simulink model "ES106A_StHlthSigStc"  (R2013b)
settings: Solver=FixedStepDiscrete  SolverMode=SingleTasking  StartTime=0.0  StopTime=1  FixedStep=0.002  RelTol=1e-3
undefined symbols (not defined in the file): APPL10_CNT_U08, BITSPERBYTE_CNT_U08, ENOTOK_CNT_U08, EOK_CNT_U08, LOWRMASKVAL_CNT_U32, NROFCRCAREA_CNT_U08, NVMAVRGPOSN_CNT_U08, NvmGetErrSts1, NVMMAXPOSN_CNT_U08, NVMMINPOSN_CNT_U08, NVMSAMPLECNTRPOSN_CNT_U08, RAMMAXPOSN_CNT_U08, RAMMINPOSN_CNT_U08, RAMRAWPOSN_CNT_U08, SIGCNT_ULS_U08, SigStcPrmInst, STHLTHMAXVAL_CNT_U08, STHLTHOSAPPL_CNT_U16, StHlthTaskRef1, WORDSIZE_CNT_U08
libraries: simulink x43, NxtrNvM x4, NxtrMax x4, NxtrMin x4, FloatToFixd x3, NxtrLim x2
(part 2 of 5)

== system ES106A_StHlthSigStc/StHlthSigStc/StHlthSigStcInit1/Check Applicability ==
  CalCRC8 : Inport
  Action Port : ActionPort  ActionType=then
  "Applicablity Check " : If  IfExpression=u1 == 1
  Constant : Constant  RequirementInfo={'linktype_rmi_doors' '0001022b (/ESG Group/FDD Module Requirements/EA4 Specific/ES106A_StHlthSigStc )' '#ES106A_48' 'true' 'REQ:ES106A_48' '' } %GIDa_4df2eb89_9649_4240_9516_a969529fb5fc  Value=0  OutDataTypeStr=uint8
      settings: AttributesFormatString=%<OutDataTypeStr>
  Data Store Read : DataStoreRead  DataStoreName=SigStcHistDataAry
  Do Nothing : Subsystem  TreatAsAtomicUnit=on
  Relational Operator : RelationalOperator  RequirementInfo={'linktype_rmi_doors' '0001022b (/ESG Group/FDD Module Requirements/EA4 Specific/ES106A_StHlthSigStc )' '#ES106A_50' 'true' 'REQ:ES106A_50' '' } %GIDa_be62b0a0_e56f_4259_a403_214fd52265b6  Operator=~=  OutDataTypeStr=boolean
  Selector : Selector  IndexMode=Zero-based  InputPortWidth=225  IndexOptions=Starting index (port)  Indices=[1 3]  OutputSizes=1
  Set Nvm Invalid : Subsystem  RequirementInfo={'linktype_rmi_doors' '0001022b (/ESG Group/FDD Module Requirements/EA4 Specific/ES106A_StHlthSigStc )' '#ES106A_44' 'true' 'REQ:ES106A_44' '' ; 'linktype_rmi_doors' '0001022b (/ESG Group/FDD Module Requirements/EA4 Specific/ES106A_StHlthSigStc )' '#ES106A_50' 'true' 'REQ:ES106A_50' '' } %GIDa_d83f31c6_88cf_451f_bc3f_a437a61baf7f  TreatAsAtomicUnit=on
  Subsystem5 : Subsystem  Description=|  mask(Copyright Information){none=on}
      | Copyright info block.                                               
      |                                                                     
      | Place copyright information at the top of every subsystem in design.
      mask prompts: none "No parameters"
      mask help: Place copyright information at the top of every subsystem in design.
      mask Display:
      | NxtrConf = 'Nexteer Confidential';
      | 
      | sys = bdroot; %handle for the current model ("system")
      | first = get_param(sys,'Created');
      | first = first(end-3:end);  %year is last four digits
      | 
      | last = get_param(sys,'LastModifiedDate');
      | if isempty(last)
      |     last = datestr(now,'yyyy');
      | else
      |     last = last(end-3:end);
      | end
      | 
      | if strcmp(first,last)
      |     fprintf('%s -- Copyright %s Nexteer',NxtrConf,first)
      | else
      |     fprintf('%s -- %s%s- %s Nexteer',NxtrConf,char(169),first,last)
      | end
  wires:
  CalCRC8/1 -> Relational Operator/2
  Relational Operator/1 -> "Applicablity Check "/1
  "Applicablity Check "/1 -> Set Nvm Invalid/Action
  "Applicablity Check "/2 -> Do Nothing/Action
  Data Store Read/1 -> Selector/1
  Constant/1 -> Selector/2
  Selector/1 -> Relational Operator/1

== system ES106A_StHlthSigStc/StHlthSigStc/StHlthSigStcInit1/CopyRight2 ==

== system ES106A_StHlthSigStc/StHlthSigStc/StHlthSigStcInit1/Crc_CalculateCRC8 ==
  note: This is the block representing the client call
  Crc_DataPtr : Inport
  Crc_Length : Inport  Port=2
  Crc_StartValue8 : Inport  Port=3
  Crc_IsFirstCall : Inport  Port=4
  Copyright1 : Subsystem  Description=|  mask(Copyright Information){none=on}
      | Copyright info block.                                               
      |                                                                     
      | Place copyright information at the top of every subsystem in design.
      mask prompts: none "No parameters"
      mask help: Place copyright information at the top of every subsystem in design.
      mask Display:
      | NxtrConf = 'Nexteer Confidential';
      | 
      | sys = bdroot; %handle for the current model ("system")
      | first = get_param(sys,'Created');
      | if(isempty(first))
      |     first = datestr(now,'yyyy');
      | else
      |     first = first(end-3:end);  %year is last four digits
      | end
      | 
      | last = get_param(sys,'LastModifiedDate');
      | if isempty(last)
      |     last = datestr(now,'yyyy');
      | else
      |     last = last(end-3:end);
      | end
      | 
      | if strcmp(first,last)
      |     fprintf('%s\nCopyright  %s Nexteer',NxtrConf,first);
      | else
      |     fprintf('%s\n%s%s-%s Nexteer',NxtrConf,char(169),first,last);
      | end
  FirstCall = False1 : Constant  Value=0  OutDataTypeStr=uint8
      settings: AttributesFormatString=%<OutDataTypeStr>
  FirstCall = False2 : Constant  Value=0  OutDataTypeStr=uint8
      settings: AttributesFormatString=%<OutDataTypeStr>
  Selector : Selector  IndexMode=Zero-based  InputPortWidth=32  IndexOptions=Starting index (port)  Indices=[1 3]  OutputSizes=1
  Terminator{1..4} (4 alike) : Terminator
  CalCRC8 : Outport
  wires:
  Crc_Length/1 -> Terminator1/1
  Crc_StartValue8/1 -> Terminator2/1
  Crc_IsFirstCall/1 -> Terminator3/1
  FirstCall = False1/1 -> CalCRC8/1
  Crc_DataPtr/1 -> Selector/1
  Selector/1 -> Terminator4/1
  FirstCall = False2/1 -> Selector/2

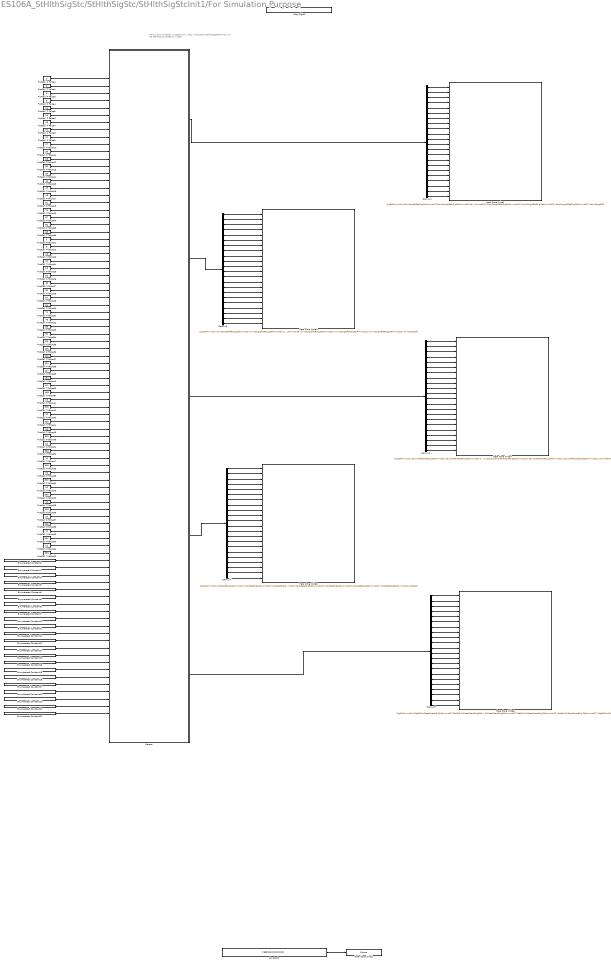
== system ES106A_StHlthSigStc/StHlthSigStc/StHlthSigStcInit1/For Simulation Purpose ==
  note: This is for Simulation purpose only.
      | Array of stucture 'StHlthSigStcPrmInst' will be defined as constant in code
  Constant9 : Constant  Description=[DUMMYAPPLCRC_CNT_U32 DUMMYCALL1CRC_CNT_U32 DUMMYCAL2CRC_CNT_U32 0 0 0 0 0]  Value=[100 10 0 0 0 0 0 0]  OutDataTypeStr=uint32
      settings: AttributesFormatString=%<Description>
  CopyRight2 : Subsystem  Description=|  mask(Copyright Information){none=on}
      | Copyright info block.                                               
      |                                                                     
      | Place copyright information at the top of every subsystem in design.
      mask prompts: none "No parameters"
      mask help: Place copyright information at the top of every subsystem in design.
      mask Display:
      | NxtrConf = 'Nexteer Confidential';
      | 
      | sys = bdroot; %handle for the current model ("system")
      | first = get_param(sys,'Created');
      | first = first(end-3:end);  %year is last four digits
      | 
      | last = get_param(sys,'LastModifiedDate');
      | if isempty(last)
      |     last = datestr(now,'yyyy');
      | else
      |     last = last(end-3:end);
      | end
      | 
      | if strcmp(first,last)
      |     fprintf('%s -- Copyright %s Nexteer',NxtrConf,first)
      | else
      |     fprintf('%s -- %s%s- %s Nexteer',NxtrConf,char(169),first,last)
      | end
  Data Store Write1 : DataStoreWrite  DataStoreName=CrcInst
  Data Store Write2 : DataStoreWrite  DataStoreName=SigStcPrmInst  DataStoreElements=SigStcPrmInst(1).RamStorgOffs#SigStcPrmInst(2).RamStorgOffs#SigStcPrmInst(3).RamStorgOffs#SigStcPrmInst(4).RamStorgOffs#SigStcPrmInst(5).RamStorgOffs#SigStcPrmInst(6).RamStorgOffs#SigStcPrmInst(7).RamStorgOffs#SigStcPrmInst(8).RamStorgOffs#SigStcPrmInst(9).RamStorgOffs#SigStcPrmInst(10).RamStorgOffs#SigStcPrmInst(11).RamStorgOffs#SigStcPrmInst(12).RamStorgOffs#SigStcPrmInst(13).RamStorgOffs#SigStcPrmInst(14).RamStorgOffs#SigStcPrmInst(15).RamStorgOffs#SigStcPrmInst(16).RamStorgOffs#SigStcPrmInst(17).RamStorgOffs#SigStcPrmInst(18).RamStorgOffs#SigStcPrmInst(19).RamStorgOffs#SigStcPrmInst(20).RamStorgOffs#SigStcPrmInst(21).RamStorgOffs#SigStcPrmInst(22).RamStorgOffs
  Data Store Write3 : DataStoreWrite  DataStoreName=SigStcPrmInst  DataStoreElements=SigStcPrmInst(1).NvmStorgOffs#SigStcPrmInst(2).NvmStorgOffs#SigStcPrmInst(3).NvmStorgOffs#SigStcPrmInst(4).NvmStorgOffs#SigStcPrmInst(5).NvmStorgOffs#SigStcPrmInst(6).NvmStorgOffs#SigStcPrmInst(7).NvmStorgOffs#SigStcPrmInst(8).NvmStorgOffs#SigStcPrmInst(9).NvmStorgOffs#SigStcPrmInst(10).NvmStorgOffs#SigStcPrmInst(11).NvmStorgOffs#SigStcPrmInst(12).NvmStorgOffs#SigStcPrmInst(13).NvmStorgOffs#SigStcPrmInst(14).NvmStorgOffs#SigStcPrmInst(15).NvmStorgOffs#SigStcPrmInst(16).NvmStorgOffs#SigStcPrmInst(17).NvmStorgOffs#SigStcPrmInst(18).NvmStorgOffs#SigStcPrmInst(19).NvmStorgOffs#SigStcPrmInst(20).NvmStorgOffs#SigStcPrmInst(21).NvmStorgOffs#SigStcPrmInst(22).NvmStorgOffs
  Data Store Write4 : DataStoreWrite  DataStoreName=SigStcPrmInst  DataStoreElements=SigStcPrmInst(1).SamplePerSec#SigStcPrmInst(2).SamplePerSec#SigStcPrmInst(3).SamplePerSec#SigStcPrmInst(4).SamplePerSec#SigStcPrmInst(5).SamplePerSec#SigStcPrmInst(6).SamplePerSec#SigStcPrmInst(7).SamplePerSec#SigStcPrmInst(8).SamplePerSec#SigStcPrmInst(9).SamplePerSec#SigStcPrmInst(10).SamplePerSec#SigStcPrmInst(11).SamplePerSec#SigStcPrmInst(12).SamplePerSec#SigStcPrmInst(13).SamplePerSec#SigStcPrmInst(14).SamplePerSec#SigStcPrmInst(15).SamplePerSec#SigStcPrmInst(16).SamplePerSec#SigStcPrmInst(17).SamplePerSec#SigStcPrmInst(18).SamplePerSec#SigStcPrmInst(19).SamplePerSec#SigStcPrmInst(20).SamplePerSec#SigStcPrmInst(21).SamplePerSec#SigStcPrmInst(22).SamplePerSec
  Data Store Write5 : DataStoreWrite  DataStoreName=SigStcPrmInst  DataStoreElements=SigStcPrmInst(1).TaskRef#SigStcPrmInst(2).TaskRef#SigStcPrmInst(3).TaskRef#SigStcPrmInst(4).TaskRef#SigStcPrmInst(5).TaskRef#SigStcPrmInst(6).TaskRef#SigStcPrmInst(7).TaskRef#SigStcPrmInst(8).TaskRef#SigStcPrmInst(9).TaskRef#SigStcPrmInst(10).TaskRef#SigStcPrmInst(11).TaskRef#SigStcPrmInst(12).TaskRef#SigStcPrmInst(13).TaskRef#SigStcPrmInst(14).TaskRef#SigStcPrmInst(15).TaskRef#SigStcPrmInst(16).TaskRef#SigStcPrmInst(17).TaskRef#SigStcPrmInst(18).TaskRef#SigStcPrmInst(19).TaskRef#SigStcPrmInst(20).TaskRef#SigStcPrmInst(21).TaskRef#SigStcPrmInst(22).TaskRef
  Data Store Write6 : DataStoreWrite  DataStoreName=SigStcPrmInst  DataStoreElements=SigStcPrmInst(1).GetStHlthDataOper#SigStcPrmInst(2).GetStHlthDataOper#SigStcPrmInst(3).GetStHlthDataOper#SigStcPrmInst(4).GetStHlthDataOper#SigStcPrmInst(5).GetStHlthDataOper#SigStcPrmInst(6).GetStHlthDataOper#SigStcPrmInst(7).GetStHlthDataOper#SigStcPrmInst(8).GetStHlthDataOper#SigStcPrmInst(9).GetStHlthDataOper#SigStcPrmInst(10).GetStHlthDataOper#SigStcPrmInst(11).GetStHlthDataOper#SigStcPrmInst(12).GetStHlthDataOper#SigStcPrmInst(13).GetStHlthDataOper#SigStcPrmInst(14).GetStHlthDataOper#SigStcPrmInst(15).GetStHlthDataOper#SigStcPrmInst(16).GetStHlthDataOper#SigStcPrmInst(17).GetStHlthDataOper#SigStcPrmInst(18).GetStHlthDataOper#SigStcPrmInst(19).GetStHlthDataOper#SigStcPrmInst(20).GetStHlthDataOper#SigStcPrmInst(21).GetStHlthDataOper#SigStcPrmInst(22).GetStHlthDataOper
  Demux{1..3,7..8} (5 alike) : Demux  Outputs=22
  Enumerated Constant{1,3,5,7,9,11,13,15,17,19,21} (11 alike) : simulink/Sources/Enumerated Constant  OutDataTypeStr=Enum: StHlthTaskRef1  Value=StHlthTaskRef1.Task_2ms_Appl10  SampleTime=inf
  Enumerated Constant{2,4,6,8,10,12,14,16,18,20,22} (11 alike) : simulink/Sources/Enumerated Constant  OutDataTypeStr=Enum: StHlthTaskRef1  Value=StHlthTaskRef1.Task_100ms_Appl10  SampleTime=inf
  FirstCall = False1 : Constant  Value=3  OutDataTypeStr=uint8
      settings: AttributesFormatString=%<OutDataTypeStr>
  FirstCall = False10 : Constant  Value=27  OutDataTypeStr=uint8
      settings: AttributesFormatString=%<OutDataTypeStr>
  FirstCall = False11 : Constant  Value=30  OutDataTypeStr=uint8
      settings: AttributesFormatString=%<OutDataTypeStr>
  FirstCall = False12 : Constant  Value=33  OutDataTypeStr=uint8
      settings: AttributesFormatString=%<OutDataTypeStr>
  FirstCall = False13 : Constant  Value=36  OutDataTypeStr=uint8
      settings: AttributesFormatString=%<OutDataTypeStr>
  FirstCall = False14 : Constant  Value=39  OutDataTypeStr=uint8
      settings: AttributesFormatString=%<OutDataTypeStr>
  FirstCall = False15 : Constant  Value=42  OutDataTypeStr=uint8
      settings: AttributesFormatString=%<OutDataTypeStr>
  FirstCall = False16 : Constant  Value=45  OutDataTypeStr=uint8
      settings: AttributesFormatString=%<OutDataTypeStr>
  FirstCall = False17 : Constant  Value=48  OutDataTypeStr=uint8
      settings: AttributesFormatString=%<OutDataTypeStr>
  FirstCall = False18 : Constant  Value=51  OutDataTypeStr=uint8
      settings: AttributesFormatString=%<OutDataTypeStr>
  FirstCall = False19 : Constant  Value=54  OutDataTypeStr=uint8
      settings: AttributesFormatString=%<OutDataTypeStr>
  FirstCall = False2 : Constant  Value=0  OutDataTypeStr=uint8
      settings: AttributesFormatString=%<OutDataTypeStr>
  FirstCall = False20 : Constant  Value=57  OutDataTypeStr=uint8
      settings: AttributesFormatString=%<OutDataTypeStr>
  FirstCall = False21 : Constant  OutDataTypeStr=uint8
      settings: AttributesFormatString=%<OutDataTypeStr>
  FirstCall = False22 : Constant  Value=8  OutDataTypeStr=uint8
      settings: AttributesFormatString=%<OutDataTypeStr>
  FirstCall = False23 : Constant  Value=15  OutDataTypeStr=uint8
      settings: AttributesFormatString=%<OutDataTypeStr>
  FirstCall = False24 : Constant  Value=22  OutDataTypeStr=uint8
      settings: AttributesFormatString=%<OutDataTypeStr>
  FirstCall = False25 : Constant  Value=29  OutDataTypeStr=uint8
      settings: AttributesFormatString=%<OutDataTypeStr>
  FirstCall = False26 : Constant  Value=36  OutDataTypeStr=uint8
      settings: AttributesFormatString=%<OutDataTypeStr>
  FirstCall = False27 : Constant  Value=43  OutDataTypeStr=uint8
      settings: AttributesFormatString=%<OutDataTypeStr>
  FirstCall = False28 : Constant  Value=50  OutDataTypeStr=uint8
      settings: AttributesFormatString=%<OutDataTypeStr>
  FirstCall = False29 : Constant  Value=57  OutDataTypeStr=uint8
      settings: AttributesFormatString=%<OutDataTypeStr>
  FirstCall = False3 : Constant  Value=6  OutDataTypeStr=uint8
      settings: AttributesFormatString=%<OutDataTypeStr>
  FirstCall = False30 : Constant  Value=64  OutDataTypeStr=uint8
      settings: AttributesFormatString=%<OutDataTypeStr>
  FirstCall = False31 : Constant  Value=71  OutDataTypeStr=uint8
      settings: AttributesFormatString=%<OutDataTypeStr>
  FirstCall = False32 : Constant  Value=78  OutDataTypeStr=uint8
      settings: AttributesFormatString=%<OutDataTypeStr>
  FirstCall = False33 : Constant  Value=85  OutDataTypeStr=uint8
      settings: AttributesFormatString=%<OutDataTypeStr>
  FirstCall = False34 : Constant  Value=92  OutDataTypeStr=uint8
      settings: AttributesFormatString=%<OutDataTypeStr>
  FirstCall = False35 : Constant  Value=99  OutDataTypeStr=uint8
      settings: AttributesFormatString=%<OutDataTypeStr>
  FirstCall = False36 : Constant  Value=106  OutDataTypeStr=uint8
      settings: AttributesFormatString=%<OutDataTypeStr>
  FirstCall = False37 : Constant  Value=113  OutDataTypeStr=uint8
      settings: AttributesFormatString=%<OutDataTypeStr>
  FirstCall = False38 : Constant  Value=120  OutDataTypeStr=uint8
      settings: AttributesFormatString=%<OutDataTypeStr>
  FirstCall = False39 : Constant  Value=127  OutDataTypeStr=uint8
      settings: AttributesFormatString=%<OutDataTypeStr>
  FirstCall = False4 : Constant  Value=9  OutDataTypeStr=uint8
      settings: AttributesFormatString=%<OutDataTypeStr>
  FirstCall = False40 : Constant  Value=134  OutDataTypeStr=uint8
      settings: AttributesFormatString=%<OutDataTypeStr>
  FirstCall = False{41,43,45,47,49,51,53,55,57,59,61} (11 alike) : Constant  Value=10  OutDataTypeStr=uint16
      settings: AttributesFormatString=%<OutDataTypeStr>
  FirstCall = False{42,44,46,48,50,52,54,56,58,60,62} (11 alike) : Constant  Value=500  OutDataTypeStr=uint16
      settings: AttributesFormatString=%<OutDataTypeStr>
  FirstCall = False5 : Constant  Value=12  OutDataTypeStr=uint8
      settings: AttributesFormatString=%<OutDataTypeStr>
  FirstCall = False6 : Constant  Value=15  OutDataTypeStr=uint8
      settings: AttributesFormatString=%<OutDataTypeStr>
  FirstCall = False63 : Constant  Value=141  OutDataTypeStr=uint8
      settings: AttributesFormatString=%<OutDataTypeStr>
  FirstCall = False64 : Constant  Value=148  OutDataTypeStr=uint8
      settings: AttributesFormatString=%<OutDataTypeStr>
  FirstCall = False65 : Constant  Value=60  OutDataTypeStr=uint8
      settings: AttributesFormatString=%<OutDataTypeStr>
  FirstCall = False66 : Constant  Value=63  OutDataTypeStr=uint8
      settings: AttributesFormatString=%<OutDataTypeStr>
  FirstCall = False7 : Constant  Value=18  OutDataTypeStr=uint8
      settings: AttributesFormatString=%<OutDataTypeStr>
  FirstCall = False8 : Constant  Value=21  OutDataTypeStr=uint8
      settings: AttributesFormatString=%<OutDataTypeStr>
  FirstCall = False9 : Constant  Value=24  OutDataTypeStr=uint8
      settings: AttributesFormatString=%<OutDataTypeStr>
  Merger : Subsystem
  wires:
  Constant9/1 -> Data Store Write1/1
  FirstCall = False2/1 -> Merger/1(RamOffs1)
  FirstCall = False1/1 -> Merger/2(RamOffs2)
  FirstCall = False3/1 -> Merger/3(RamOffs3)
  FirstCall = False4/1 -> Merger/4(RamOffs4)
  FirstCall = False5/1 -> Merger/5(RamOffs5)
  FirstCall = False6/1 -> Merger/6(RamOffs6)
  FirstCall = False7/1 -> Merger/7(RamOffs7)
  FirstCall = False8/1 -> Merger/8(RamOffs8)
  FirstCall = False9/1 -> Merger/9(RamOffs9)
  FirstCall = False10/1 -> Merger/10(RamOffs10)
  FirstCall = False11/1 -> Merger/11(RamOffs11)
  FirstCall = False12/1 -> Merger/12(RamOffs17)
  FirstCall = False14/1 -> Merger/14(RamOffs13)
  FirstCall = False15/1 -> Merger/15(RamOffs14)
  FirstCall = False16/1 -> Merger/16(RamOffs15)
  FirstCall = False17/1 -> Merger/17(RamOffs16)
  FirstCall = False18/1 -> Merger/18(RamOffs18)
  FirstCall = False19/1 -> Merger/19(RamOffs19)
  FirstCall = False20/1 -> Merger/20(RamOffs20)
  FirstCall = False21/1 -> Merger/23(NVMOffs1)
  FirstCall = False22/1 -> Merger/24(NVMOffs2)
  FirstCall = False23/1 -> Merger/25(NVMOffs3)
  FirstCall = False24/1 -> Merger/26(NVMOffs4)
  FirstCall = False25/1 -> Merger/27(NVMOffs5)
  FirstCall = False26/1 -> Merger/28(NVMOffs6)
  FirstCall = False27/1 -> Merger/29(NVMOffs7)
  FirstCall = False28/1 -> Merger/30(NVMOffs8)
  FirstCall = False29/1 -> Merger/31(NVMOffs9)
  FirstCall = False30/1 -> Merger/32(NVMOffs10)
  FirstCall = False31/1 -> Merger/33(NVMOffs11)
  FirstCall = False32/1 -> Merger/34(NVMOffs12)
  FirstCall = False33/1 -> Merger/35(NVMOffs13)
  FirstCall = False34/1 -> Merger/36(NVMOffs14)
  FirstCall = False35/1 -> Merger/37(NVMOffs15)
  FirstCall = False36/1 -> Merger/38(NVMOffs16)
  FirstCall = False37/1 -> Merger/39(NVMOffs17)
  FirstCall = False38/1 -> Merger/40(NVMOffs18)
  FirstCall = False39/1 -> Merger/41(NVMOffs19)
  FirstCall = False40/1 -> Merger/42(NVMOffs20)
  FirstCall = False41/1 -> Merger/45(SamplePerSec1)
  FirstCall = False42/1 -> Merger/46(SamplePerSec2)
  Enumerated Constant2/1 -> Merger/67(TaskRef1)
  Enumerated Constant1/1 -> Merger/68(TaskRef2)
  FirstCall = False13/1 -> Merger/13(RamOffs12)
  Merger/2(NVMOffs23) -> Demux3/1
  Demux3/7 -> Data Store Write3/7
  Demux3/9 -> Data Store Write3/9
  Demux3/8 -> Data Store Write3/8
  Demux3/12 -> Data Store Write3/12
  Demux3/11 -> Data Store Write3/11
  Demux3/14 -> Data Store Write3/14
  Demux3/15 -> Data Store Write3/15
  Demux3/16 -> Data Store Write3/16
  Demux3/19 -> Data Store Write3/19
  Demux3/18 -> Data Store Write3/18
  Demux3/20 -> Data Store Write3/20
  Demux3/10 -> Data Store Write3/10
  Demux3/13 -> Data Store Write3/13
  Demux3/2 -> Data Store Write3/2
  Demux3/4 -> Data Store Write3/4
  Demux3/17 -> Data Store Write3/17
  Demux3/5 -> Data Store Write3/5
  Demux3/6 -> Data Store Write3/6
  Demux3/1 -> Data Store Write3/1
  Demux3/3 -> Data Store Write3/3
  Demux7/2 -> Data Store Write5/2
  Demux7/1 -> Data Store Write5/1
  Merger/4(TaskRef) -> Demux7/1
  Demux7/16 -> Data Store Write5/16
  Demux7/12 -> Data Store Write5/12
  Demux7/3 -> Data Store Write5/3
  Demux7/11 -> Data Store Write5/11
  Demux7/19 -> Data Store Write5/19
  Demux7/9 -> Data Store Write5/9
  Demux7/18 -> Data Store Write5/18
  Demux7/17 -> Data Store Write5/17
  Demux7/20 -> Data Store Write5/20
  Demux7/6 -> Data Store Write5/6
  Demux7/4 -> Data Store Write5/4
  Demux7/5 -> Data Store Write5/5
  Demux7/7 -> Data Store Write5/7
  Demux7/13 -> Data Store Write5/13
  Demux7/15 -> Data Store Write5/15
  Demux7/10 -> Data Store Write5/10
  Demux7/14 -> Data Store Write5/14
  Demux7/8 -> Data Store Write5/8
  Demux8/2 -> Data Store Write6/2
  Demux8/1 -> Data Store Write6/1
  Demux8/3 -> Data Store Write6/3
  Merger/5(GetOper) -> Demux8/1
  Demux8/4 -> Data Store Write6/4
  Demux8/18 -> Data Store Write6/18
  Demux8/17 -> Data Store Write6/17
  Demux8/5 -> Data Store Write6/5
  Demux8/9 -> Data Store Write6/9
  Demux8/15 -> Data Store Write6/15
  Demux8/13 -> Data Store Write6/13
  Demux8/14 -> Data Store Write6/14
  Demux8/19 -> Data Store Write6/19
  Demux8/7 -> Data Store Write6/7
  Demux8/11 -> Data Store Write6/11
  Demux8/6 -> Data Store Write6/6
  Demux8/20 -> Data Store Write6/20
  Demux8/16 -> Data Store Write6/16
  Demux8/8 -> Data Store Write6/8
  Demux8/12 -> Data Store Write6/12
  Demux8/10 -> Data Store Write6/10
  Demux1/2 -> Data Store Write2/2
  Demux1/1 -> Data Store Write2/1
  Merger/1(RamOffs) -> Demux1/1
  Demux1/6 -> Data Store Write2/6
  Demux1/12 -> Data Store Write2/12
  Demux1/5 -> Data Store Write2/5
  Demux1/10 -> Data Store Write2/10
  Demux1/18 -> Data Store Write2/18
  Demux1/9 -> Data Store Write2/9
  Demux1/4 -> Data Store Write2/4
  Demux1/8 -> Data Store Write2/8
  Demux1/7 -> Data Store Write2/7
  Demux1/11 -> Data Store Write2/11
  Demux1/3 -> Data Store Write2/3
  Demux1/19 -> Data Store Write2/19
  Demux1/15 -> Data Store Write2/15
  Demux1/16 -> Data Store Write2/16
  Demux1/14 -> Data Store Write2/14
  Demux1/17 -> Data Store Write2/17
  Demux1/20 -> Data Store Write2/20
  Demux1/13 -> Data Store Write2/13
  Demux2/1 -> Data Store Write4/1
  Demux2/2 -> Data Store Write4/2
  Demux2/3 -> Data Store Write4/3
  Demux2/4 -> Data Store Write4/4
  Demux2/5 -> Data Store Write4/5
  Demux2/6 -> Data Store Write4/6
  Demux2/7 -> Data Store Write4/7
  Demux2/8 -> Data Store Write4/8
  Demux2/9 -> Data Store Write4/9
  Demux2/10 -> Data Store Write4/10
  Demux2/11 -> Data Store Write4/11
  Demux2/12 -> Data Store Write4/12
  Demux2/13 -> Data Store Write4/13
  Demux2/14 -> Data Store Write4/14
  Demux2/15 -> Data Store Write4/15
  Demux2/16 -> Data Store Write4/16
  Demux2/17 -> Data Store Write4/17
  Demux2/18 -> Data Store Write4/18
  Demux2/19 -> Data Store Write4/19
  Demux2/20 -> Data Store Write4/20
  Merger/3(SampelPersec1) -> Demux2/1
  FirstCall = False44/1 -> Merger/48(SamplePerSec4)
  FirstCall = False43/1 -> Merger/47(SamplePerSec3)
  FirstCall = False45/1 -> Merger/49(SamplePerSec5)
  FirstCall = False46/1 -> Merger/50(SamplePerSec6)
  FirstCall = False51/1 -> Merger/51(SamplePerSec7)
  FirstCall = False52/1 -> Merger/52(SamplePerSec8)
  FirstCall = False47/1 -> Merger/53(SamplePerSec9)
  FirstCall = False48/1 -> Merger/54(SamplePerSec10)
  FirstCall = False53/1 -> Merger/55(SamplePerSec11)
  FirstCall = False54/1 -> Merger/56(SamplePerSec12)
  FirstCall = False50/1 -> Merger/58(SamplePerSec14)
  FirstCall = False49/1 -> Merger/57(SamplePerSec13)
  FirstCall = False55/1 -> Merger/59(SamplePerSec15)
  FirstCall = False56/1 -> Merger/60(SamplePerSec16)
  FirstCall = False58/1 -> Merger/62(SamplePerSec18)
  FirstCall = False57/1 -> Merger/61(SamplePerSec17)
  FirstCall = False60/1 -> Merger/64(SamplePerSec20)
  FirstCall = False59/1 -> Merger/63(SamplePerSec19)
  Enumerated Constant3/1 -> Merger/70(TaskRef4)
  Enumerated Constant4/1 -> Merger/69(TaskRef3)
  Enumerated Constant5/1 -> Merger/72(TaskRef6)
  Enumerated Constant6/1 -> Merger/71(TaskRef5)
  Enumerated Constant7/1 -> Merger/74(TaskRef8)
  Enumerated Constant8/1 -> Merger/73(TaskRef7)
  Enumerated Constant9/1 -> Merger/76(TaskRef10)
  Enumerated Constant10/1 -> Merger/75(TaskRef9)
  Enumerated Constant11/1 -> Merger/78(TaskRef12)
  Enumerated Constant12/1 -> Merger/77(TaskRef11)
  Enumerated Constant14/1 -> Merger/79(TaskRef13)
  Enumerated Constant13/1 -> Merger/80(TaskRef14)
  Enumerated Constant16/1 -> Merger/81(TaskRef15)
  Enumerated Constant15/1 -> Merger/82(TaskRef16)
  Enumerated Constant20/1 -> Merger/85(TaskRef19)
  Enumerated Constant19/1 -> Merger/86(TaskRef20)
  Enumerated Constant18/1 -> Merger/83(TaskRef17)
  Enumerated Constant17/1 -> Merger/84(TaskRef18)
  Demux1/21 -> Data Store Write2/21
  Demux1/22 -> Data Store Write2/22
  Demux3/21 -> Data Store Write3/21
  Demux3/22 -> Data Store Write3/22
  Demux2/21 -> Data Store Write4/21
  Demux2/22 -> Data Store Write4/22
  Demux7/21 -> Data Store Write5/21
  Demux7/22 -> Data Store Write5/22
  Demux8/21 -> Data Store Write6/21
  Demux8/22 -> Data Store Write6/22
  FirstCall = False65/1 -> Merger/21(RamOffs21)
  FirstCall = False66/1 -> Merger/22(RamOffs22)
  FirstCall = False64/1 -> Merger/44(NVMOffs22)
  FirstCall = False63/1 -> Merger/43(NVMOffs21)
  FirstCall = False62/1 -> Merger/66(SamplePerSec22)
  FirstCall = False61/1 -> Merger/65(SamplePerSec21)
  Enumerated Constant21/1 -> Merger/88(TaskRef22)
  Enumerated Constant22/1 -> Merger/87(TaskRef21)

== system ES106A_StHlthSigStc/StHlthSigStc/StHlthSigStcInit1/Initialize Nvm ==
  CalCRC8 : Inport
  Action Port : ActionPort  ActionType=then
  Assignment : Assignment  IndexMode=Zero-based  IndexOptions=Index vector (port)  Indices=1  OutputSizes=1
  Constant1 : Constant  Value=0  OutDataTypeStr=uint8
      settings: AttributesFormatString=%<OutDataTypeStr>
  Constant2 : Constant  Value=0*(1:225)  OutDataTypeStr=uint8
      settings: AttributesFormatString=%<OutDataTypeStr>
  Data Store Read1 : DataStoreRead  DataStoreName=SigStcHistDataAry
  Data Store Write : DataStoreWrite  DataStoreName=SigStcHistDataAry
  Data Store Write1 : DataStoreWrite  DataStoreName=SigStcHistDataAry
  Subsystem5 : Subsystem  Description=|  mask(Copyright Information){none=on}
      | Copyright info block.                                               
      |                                                                     
      | Place copyright information at the top of every subsystem in design.
      mask prompts: none "No parameters"
      mask help: Place copyright information at the top of every subsystem in design.
      mask Display:
      | NxtrConf = 'Nexteer Confidential';
      | 
      | sys = bdroot; %handle for the current model ("system")
      | first = get_param(sys,'Created');
      | first = first(end-3:end);  %year is last four digits
      | 
      | last = get_param(sys,'LastModifiedDate');
      | if isempty(last)
      |     last = datestr(now,'yyyy');
      | else
      |     last = last(end-3:end);
      | end
      | 
      | if strcmp(first,last)
      |     fprintf('%s -- Copyright %s Nexteer',NxtrConf,first)
      | else
      |     fprintf('%s -- %s%s- %s Nexteer',NxtrConf,char(169),first,last)
      | end
  wires:
  Data Store Read1/1 -> Assignment/1
  Constant1/1 -> Assignment/3
  CalCRC8/1 -> Assignment/2
  Assignment/1 -> Data Store Write/1
  Constant2/1 -> Data Store Write1/1

== system ES106A_StHlthSigStc/StHlthSigStc/StHlthSigStcInit1/Initialize the Minimum value for all SOH signals ==
  SigCnt : Inport
  Add : Sum
  Assignment : Assignment  IndexMode=Zero-based  IndexOptions=Index vector (port)  Indices=1  OutputSizes=1
  Bus Selector2 : BusSelector  OutputSignals=RamStorgOffs
  Constant : Constant  Value=RAMMINPOSN_CNT_U08
  Constant1 : Constant  Value=STHLTHMAXVAL_CNT_U08  OutDataTypeStr=uint8
      settings: AttributesFormatString=%<OutDataTypeStr>
  Data Store Read : DataStoreRead  DataStoreName=RamBuf
  Data Store Read6 : DataStoreRead  DataStoreName=SigStcPrmInst  DataStoreElements=SigStcPrmInst(:)
  Data Store Write : DataStoreWrite  DataStoreName=RamBuf
  For Iterator : ForIterator  IterationSource=external  IndexMode=Zero-based
  Selector5 : Selector  IndexMode=Zero-based  InputPortWidth=22  IndexOptions=Index vector (port)  Indices=[0 1]  OutputSizes=1
  Subsystem5 : Subsystem  Description=|  mask(Copyright Information){none=on}
      | Copyright info block.                                               
      |                                                                     
      | Place copyright information at the top of every subsystem in design.
      mask prompts: none "No parameters"
      mask help: Place copyright information at the top of every subsystem in design.
      mask Display:
      | NxtrConf = 'Nexteer Confidential';
      | 
      | sys = bdroot; %handle for the current model ("system")
      | first = get_param(sys,'Created');
      | first = first(end-3:end);  %year is last four digits
      | 
      | last = get_param(sys,'LastModifiedDate');
      | if isempty(last)
      |     last = datestr(now,'yyyy');
      | else
      |     last = last(end-3:end);
      | end
      | 
      | if strcmp(first,last)
      |     fprintf('%s -- Copyright %s Nexteer',NxtrConf,first)
      | else
      |     fprintf('%s -- %s%s- %s Nexteer',NxtrConf,char(169),first,last)
      | end
  wires:
  Assignment/1 -> Data Store Write/1
  Data Store Read/1 -> Assignment/1
  Constant/1 -> Add/1
  Constant1/1 -> Assignment/2
  Add/1 -> Assignment/3
  SigCnt/1 -> For Iterator/1
  Selector5/1 -> Bus Selector2/1
  Bus Selector2/1 -> Add/2  "<RamStorgOffs>"
  For Iterator/1 -> Selector5/2
  Data Store Read6/1 -> Selector5/1

== system ES106A_StHlthSigStc/StHlthSigStc/StHlthSigStcInit1/NvmNotVal ==
  Action Port : ActionPort  ActionType=then
  CopyRight2 : Subsystem  Description=|  mask(Copyright Information){none=on}
      | Copyright info block.                                               
      |                                                                     
      | Place copyright information at the top of every subsystem in design.
      mask prompts: none "No parameters"
      mask help: Place copyright information at the top of every subsystem in design.
      mask Display:
      | NxtrConf = 'Nexteer Confidential';
      | 
      | sys = bdroot; %handle for the current model ("system")
      | first = get_param(sys,'Created');
      | if(isempty(first))
      |     first = datestr(now,'yyyy');
      | else
      |     first = first(end-3:end);  %year is last four digits
      | end
      | 
      | last = get_param(sys,'LastModifiedDate');
      | if isempty(last)
      |     last = datestr(now,'yyyy');
      | else
      |     last = last(end-3:end);
      | end
      | 
      | if strcmp(first,last)
      |     fprintf('%s -- Copyright %s Nexteer',NxtrConf,first)
      | else
      |     fprintf('%s -- %s%s- %s Nexteer',NxtrConf,char(169),first,last)
      | end
  Data Store Write : DataStoreWrite  DataStoreName=VldNvm
  WriteFlag1 : Constant  RequirementInfo={} %GIDa_cf464d82_db66_42a8_81c0_e3b58f30b447  Value=false  OutDataTypeStr=boolean
      settings: AttributesFormatString=%<OutDataTypeStr>
  wires:
  WriteFlag1/1 -> Data Store Write/1

== system ES106A_StHlthSigStc/StHlthSigStc/StHlthSigStcInit1/Prepare a buffer for CRC calculation ==
  CopyRight2 : Subsystem  Description=|  mask(Copyright Information){none=on}
      | Copyright info block.                                               
      |                                                                     
      | Place copyright information at the top of every subsystem in design.
      mask prompts: none "No parameters"
      mask help: Place copyright information at the top of every subsystem in design.
      mask Display:
      | NxtrConf = 'Nexteer Confidential';
      | 
      | sys = bdroot; %handle for the current model ("system")
      | first = get_param(sys,'Created');
      | first = first(end-3:end);  %year is last four digits
      | 
      | last = get_param(sys,'LastModifiedDate');
      | if isempty(last)
      |     last = datestr(now,'yyyy');
      | else
      |     last = last(end-3:end);
      | end
      | 
      | if strcmp(first,last)
      |     fprintf('%s -- Copyright %s Nexteer',NxtrConf,first)
      | else
      |     fprintf('%s -- %s%s- %s Nexteer',NxtrConf,char(169),first,last)
      | end
  Data Store Read : DataStoreRead  DataStoreName=CrcInst
  FirstCall = False3 : Constant  Value=WORDSIZE_CNT_U08
  For Iterator : ForIterator  IterationLimit=2  IndexMode=Zero-based
  Iterator : Subsystem  TreatAsAtomicUnit=on
  Selector : Selector  IndexMode=Zero-based  InputPortWidth=8  IndexOptions=Starting index (port)  Indices=[1 3]  OutputSizes=1
  wires:
  For Iterator/1 -> Iterator/2(CrcOutrLoopCnt), Selector/2
  Data Store Read/1 -> Selector/1
  Selector/1 -> Iterator/1(CrcData)
  FirstCall = False3/1 -> Iterator/3(Iterator)

== system ES106A_StHlthSigStc/StHlthSigStc/StHlthStcPwrDwn/CopyRight2 ==

== system ES106A_StHlthSigStc/StHlthSigStc/StHlthStcPwrDwn/For Iterator Subsystem ==
  note: If action subsystem has been moved to above layer.
  note: SampleCnt
  SigCnt : Inport
  Bus Selector2 : BusSelector  OutputSignals=SamplePerSec,RamStorgOffs,NvmStorgOffs
  CopyRight2 : Subsystem  Description=|  mask(Copyright Information){none=on}
      | Copyright info block.                                               
      |                                                                     
      | Place copyright information at the top of every subsystem in design.
      mask prompts: none "No parameters"
      mask help: Place copyright information at the top of every subsystem in design.
      mask Display:
      | NxtrConf = 'Nexteer Confidential';
      | 
      | sys = bdroot; %handle for the current model ("system")
      | first = get_param(sys,'Created');
      | first = first(end-3:end);  %year is last four digits
      | 
      | last = get_param(sys,'LastModifiedDate');
      | if isempty(last)
      |     last = datestr(now,'yyyy');
      | else
      |     last = last(end-3:end);
      | end
      | 
      | if strcmp(first,last)
      |     fprintf('%s -- Copyright %s Nexteer',NxtrConf,first)
      | else
      |     fprintf('%s -- %s%s- %s Nexteer',NxtrConf,char(169),first,last)
      | end
  Data Store Read1 : DataStoreRead  DataStoreName=IgnCycSampleCntrAry
  Data Store Read2 : DataStoreRead  DataStoreName=SigStcPrmInst
  Divide : Product  Inputs=*/
  For Iterator : ForIterator  IterationSource=external  IterationLimit=2  IndexMode=Zero-based
  If : If  IfExpression="u1 ~=  0"  ShowElse=off
  If Action Subsystem : Subsystem  TreatAsAtomicUnit=on
  Selector : Selector  IndexMode=Zero-based  InputPortWidth=22  IndexOptions=Starting index (port)  Indices=[1 3]  OutputSizes=1
  Selector1 : Selector  IndexMode=Zero-based  InputPortWidth=22  IndexOptions=Index vector (port)  Indices=[1 3]  OutputSizes=1
  NvmWrRqrdUls : Outport
  wires:
  If/1 -> If Action Subsystem/Action
  Data Store Read2/1 -> Selector1/1
  For Iterator/1 -> If Action Subsystem/4(SigAvrgAdr), Selector/2, Selector1/2
  Selector1/1 -> Bus Selector2/1
  Selector/1 -> Divide/1
  Bus Selector2/1 -> Divide/2  "<SamplePerSec>"
  Divide/1 -> If/1, If Action Subsystem/1(SampleCnt)
  Data Store Read1/1 -> Selector/1
  Bus Selector2/2 -> If Action Subsystem/2(StrtAdr)  "<RamStorgOffs>"
  Bus Selector2/3 -> If Action Subsystem/3(NvmOffs)  "<NvmStorgOffs>"
  SigCnt/1 -> For Iterator/1
  If Action Subsystem/1(NvmWrRqrdUls) -> NvmWrRqrdUls/1

== system ES106A_StHlthSigStc/StHlthSigStc/StHlthStcPwrDwn/If Action Subsystem1 ==
  Action Port : ActionPort  ActionType=then
  Constant : Constant  Value=true  OutDataTypeStr=boolean
      settings: AttributesFormatString=%<OutDataTypeStr>
  CopyRight2 : Subsystem  Description=|  mask(Copyright Information){none=on}
      | Copyright info block.                                               
      |                                                                     
      | Place copyright information at the top of every subsystem in design.
      mask prompts: none "No parameters"
      mask help: Place copyright information at the top of every subsystem in design.
      mask Display:
      | NxtrConf = 'Nexteer Confidential';
      | 
      | sys = bdroot; %handle for the current model ("system")
      | first = get_param(sys,'Created');
      | first = first(end-3:end);  %year is last four digits
      | 
      | last = get_param(sys,'LastModifiedDate');
      | if isempty(last)
      |     last = datestr(now,'yyyy');
      | else
      |     last = last(end-3:end);
      | end
      | 
      | if strcmp(first,last)
      |     fprintf('%s -- Copyright %s Nexteer',NxtrConf,first)
      | else
      |     fprintf('%s -- %s%s- %s Nexteer',NxtrConf,char(169),first,last)
      | end
  Set Ram Block Status : NxtrNvM/Set Ram Block Status  FuncName=Set Ram Block Status  NvMBlockName=SigStcHistDataAry  VoidFuncRtn=on  BlockChanged_DSN=NvMSRBS_BlockChanged  Return_DSN=NvMSRBS_Return
      settings: AttributesFormatString=%<FuncName>
  wires:
  Constant/1 -> Set Ram Block Status/1

== system ES106A_StHlthSigStc/StHlthSigStc/UpdStHlthStcData/Call Non Trusted Function  ==
  StHlthSig : Inport
  TaskId_ArgIn : Inport  Port=2
  SigCnt : Inport  Port=3
  "Action Port " : ActionPort  ActionType=else
  CopyRight2 : Subsystem  Description=|  mask(Copyright Information){none=on}
      | Copyright info block.                                               
      |                                                                     
      | Place copyright information at the top of every subsystem in design.
      mask prompts: none "No parameters"
      mask help: Place copyright information at the top of every subsystem in design.
      mask Display:
      | NxtrConf = 'Nexteer Confidential';
      | 
      | sys = bdroot; %handle for the current model ("system")
      | first = get_param(sys,'Created');
      | if(isempty(first))
      |     first = datestr(now,'yyyy');
      | else
      |     first = first(end-3:end);  %year is last four digits
      | end
      | 
      | last = get_param(sys,'LastModifiedDate');
      | if isempty(last)
      |     last = datestr(now,'yyyy');
      | else
      |     last = last(end-3:end);
      | end
      | 
      | if strcmp(first,last)
      |     fprintf('%s -- Copyright %s Nexteer',NxtrConf,first)
      | else
      |     fprintf('%s -- %s%s- %s Nexteer',NxtrConf,char(169),first,last)
      | end
  For Iterator Subsystem : Subsystem  TreatAsAtomicUnit=on
  wires:
  TaskId_ArgIn/1 -> For Iterator Subsystem/1(TaskId_ArgIn)
  StHlthSig/1 -> For Iterator Subsystem/3(StHlthSig)
  SigCnt/1 -> For Iterator Subsystem/2(SigCnt)

== system ES106A_StHlthSigStc/StHlthSigStc/UpdStHlthStcData/CopyRight2 ==

== system ES106A_StHlthSigStc/StHlthSigStc/UpdStHlthStcData/GetApplicationID ==
  note: This client server is used to get application id of state health signal which is currently being processed.
  Constant : Constant  Value=APPL10_CNT_U08
  CopyRight2 : Subsystem  Description=|  mask(Copyright Information){none=on}
      | Copyright info block.                                               
      |                                                                     
      | Place copyright information at the top of every subsystem in design.
      mask prompts: none "No parameters"
      mask help: Place copyright information at the top of every subsystem in design.
      mask Display:
      | NxtrConf = 'Nexteer Confidential';
      | 
      | sys = bdroot; %handle for the current model ("system")
      | first = get_param(sys,'Created');
      | first = first(end-3:end);  %year is last four digits
      | 
      | last = get_param(sys,'LastModifiedDate');
      | if isempty(last)
      |     last = datestr(now,'yyyy');
      | else
      |     last = last(end-3:end);
      | end
      | 
      | if strcmp(first,last)
      |     fprintf('%s -- Copyright %s Nexteer',NxtrConf,first)
      | else
      |     fprintf('%s -- %s%s- %s Nexteer',NxtrConf,char(169),first,last)
      | end
  ApplId : Outport
  wires:
  Constant/1 -> ApplId/1

== system ES106A_StHlthSigStc/StHlthSigStc/UpdStHlthStcData/UpdDataSample ==
  StHlthSig : Inport
  TaskId_ArgIn : Inport  Port=2
  SigCnt : Inport  Port=3
  Action Port : ActionPort  ActionType=then
  CopyRight2 : Subsystem  Description=|  mask(Copyright Information){none=on}
      | Copyright info block.                                               
      |                                                                     
      | Place copyright information at the top of every subsystem in design.
      mask prompts: none "No parameters"
      mask help: Place copyright information at the top of every subsystem in design.
      mask Display:
      | NxtrConf = 'Nexteer Confidential';
      | 
      | sys = bdroot; %handle for the current model ("system")
      | first = get_param(sys,'Created');
      | if(isempty(first))
      |     first = datestr(now,'yyyy');
      | else
      |     first = first(end-3:end);  %year is last four digits
      | end
      | 
      | last = get_param(sys,'LastModifiedDate');
      | if isempty(last)
      |     last = datestr(now,'yyyy');
      | else
      |     last = last(end-3:end);
      | end
      | 
      | if strcmp(first,last)
      |     fprintf('%s -- Copyright %s Nexteer',NxtrConf,first)
      | else
      |     fprintf('%s -- %s%s- %s Nexteer',NxtrConf,char(169),first,last)
      | end
  For Iterator Subsystem : Subsystem  TreatAsAtomicUnit=on
  wires:
  TaskId_ArgIn/1 -> For Iterator Subsystem/1(TaskId_ArgIn)
  StHlthSig/1 -> For Iterator Subsystem/3(StHlthSig)
  SigCnt/1 -> For Iterator Subsystem/2(SigCnt)

== system ES106A_StHlthSigStc/StHlthSigStc/ClrSigStcHlthData/Call Non Trusted Function/Clear Nvm Data ==
  note: Clear all contents of NVM except the first byte. First byte shall remain untouched which keeps the CRC
  Action Port : ActionPort  ActionType=then
  Constant : Constant  Value=false  OutDataTypeStr=boolean
      settings: AttributesFormatString=%<OutDataTypeStr>
  Constant2 : Constant  Value=0*(1:225)  OutDataTypeStr=uint8
      settings: AttributesFormatString=%<OutDataTypeStr>
  CopyRight2 : Subsystem  Description=|  mask(Copyright Information){none=on}
      | Copyright info block.                                               
      |                                                                     
      | Place copyright information at the top of every subsystem in design.
      mask prompts: none "No parameters"
      mask help: Place copyright information at the top of every subsystem in design.
      mask Display:
      | NxtrConf = 'Nexteer Confidential';
      | 
      | sys = bdroot; %handle for the current model ("system")
      | first = get_param(sys,'Created');
      | first = first(end-3:end);  %year is last four digits
      | 
      | last = get_param(sys,'LastModifiedDate');
      | if isempty(last)
      |     last = datestr(now,'yyyy');
      | else
      |     last = last(end-3:end);
      | end
      | 
      | if strcmp(first,last)
      |     fprintf('%s -- Copyright %s Nexteer',NxtrConf,first)
      | else
      |     fprintf('%s -- %s%s- %s Nexteer',NxtrConf,char(169),first,last)
      | end
  Data Store Write1 : DataStoreWrite  DataStoreName=SigStcHistDataAry
  Data Store Write5 : DataStoreWrite  DataStoreName=VldNvm
  Set Ram Block Status : NxtrNvM/Set Ram Block Status  RequirementInfo={} %GIDa_968c04bb_e56f_48d6_8d87_8bfc99c0842a  FuncName=Set Ram Block Status  NvMBlockName=SigStcHistDataAry  VoidFuncRtn=on  BlockChanged_DSN=NvMSRBS_BlockChanged  Return_DSN=NvMSRBS_Return1
      settings: AttributesFormatString=%<FuncName>
  WriteFlag : Constant  RequirementInfo={} %GIDa_0158d9c3_2d65_4d54_880a_ae858c3e60db  Value=true  OutDataTypeStr=boolean
      settings: AttributesFormatString=%<OutDataTypeStr>
  wires:
  Constant2/1 -> Data Store Write1/1
  WriteFlag/1 -> Set Ram Block Status/1
  Constant/1 -> Data Store Write5/1

== system ES106A_StHlthSigStc/StHlthSigStc/ClrSigStcHlthData/Call Non Trusted Function/CopyRight2 ==

== system ES106A_StHlthSigStc/StHlthSigStc/ClrSigStcHlthData/Call Non Trusted Function/Dont clear Nvm Data ==
  Action Port : ActionPort  ActionType=else
  CopyRight2 : Subsystem  Description=|  mask(Copyright Information){none=on}
      | Copyright info block.                                               
      |                                                                     
      | Place copyright information at the top of every subsystem in design.
      mask prompts: none "No parameters"
      mask help: Place copyright information at the top of every subsystem in design.
      mask Display:
      | NxtrConf = 'Nexteer Confidential';
      | 
      | sys = bdroot; %handle for the current model ("system")
      | first = get_param(sys,'Created');
      | first = first(end-3:end);  %year is last four digits
      | 
      | last = get_param(sys,'LastModifiedDate');
      | if isempty(last)
      |     last = datestr(now,'yyyy');
      | else
      |     last = last(end-3:end);
      | end
      | 
      | if strcmp(first,last)
      |     fprintf('%s -- Copyright %s Nexteer',NxtrConf,first)
      | else
      |     fprintf('%s -- %s%s- %s Nexteer',NxtrConf,char(169),first,last)
      | end

== system ES106A_StHlthSigStc/StHlthSigStc/ClrSigStcHlthData/Call Non Trusted Function/For Iterator Subsystem ==
  "SigCnt " : Inport
  Add : Sum
  Assignment2 : Assignment  IndexMode=Zero-based  IndexOptions=Starting index (port)  Indices=1  OutputSizes=1
  Bus Selector2 : BusSelector  OutputSignals=RamStorgOffs
  Constant5 : Constant  Value=RAMMINPOSN_CNT_U08
  Constant6 : Constant  Value=STHLTHMAXVAL_CNT_U08  OutDataTypeStr=uint8
  CopyRight2 : Subsystem  Description=|  mask(Copyright Information){none=on}
      | Copyright info block.                                               
      |                                                                     
      | Place copyright information at the top of every subsystem in design.
      mask prompts: none "No parameters"
      mask help: Place copyright information at the top of every subsystem in design.
      mask Display:
      | NxtrConf = 'Nexteer Confidential';
      | 
      | sys = bdroot; %handle for the current model ("system")
      | first = get_param(sys,'Created');
      | first = first(end-3:end);  %year is last four digits
      | 
      | last = get_param(sys,'LastModifiedDate');
      | if isempty(last)
      |     last = datestr(now,'yyyy');
      | else
      |     last = last(end-3:end);
      | end
      | 
      | if strcmp(first,last)
      |     fprintf('%s -- Copyright %s Nexteer',NxtrConf,first)
      | else
      |     fprintf('%s -- %s%s- %s Nexteer',NxtrConf,char(169),first,last)
      | end
  Data Store Read3 : DataStoreRead  DataStoreName=SigStcPrmInst  DataStoreElements=SigStcPrmInst(:)
  Data Store Read4 : DataStoreRead  DataStoreName=RamBuf
  Data Store Write2 : DataStoreWrite  DataStoreName=RamBuf
  For Iterator : ForIterator  IterationSource=external  IndexMode=Zero-based
  Selector1 : Selector  IndexMode=Zero-based  InputPortWidth=22  IndexOptions=Index vector (port)  Indices=[1 3]  OutputSizes=1
  wires:
  "SigCnt "/1 -> For Iterator/1
  For Iterator/1 -> Selector1/2
  Selector1/1 -> Bus Selector2/1
  Data Store Read3/1 -> Selector1/1
  Bus Selector2/1 -> Add/1  "<RamStorgOffs>"
  Constant5/1 -> Add/2
  Add/1 -> Assignment2/3
  Data Store Read4/1 -> Assignment2/1
  Constant6/1 -> Assignment2/2
  Assignment2/1 -> Data Store Write2/1
